simulink model "corr_mod_2_sim41_MI"  (R2021a)
settings: Solver=ode5  StartTime=0  StopTime=3  FixedStep=0.001  MaxStep=0.01  RelTol=1e-3  AbsTol=1e-3
values from neighbouring files (symbols this model uses):
  g = 9.81    [cipendco.m]
  l = 0.36    [cipendco.m]
  m = 0.23    [cipendco.m]
  M = 2.4    [cipendco.m]
settings Model: ExtModeTrigMode=oneshot  ExtModeArmWhenConnect=off  ExtModeAutoUpdateStatusClock=off  Creator=franckplestan  LastModifiedBy=Rodrigo
settings SolverCC: AutoScaleAbsTol=off  AlgebraicLoopSolver=TrustRegion
settings DataIOCC: SaveFormat=Array  SignalLoggingSaveFormat=ModelDataLogs  SaveOutput=off  ReturnWorkspaceOutputs=off
settings OptimizationCC: BooleanDataType=off  ExpressionDepthLimit=2147483647  InitFltsAndDblsToZero=on  LifeSpan=inf
settings DebuggingCC: SaveWithParameterizedLinksMsg=none  UnderspecifiedInitializationDetection=Classic  MergeDetectMultiDrivingBlocksExec=none  SignalResolutionControl=TryResolveAllWithWarning  MultiTaskDSMMsg=warning  MultiTaskCondExecSysMsg=none  FcnCallInpInsideContextMsg=warning  StateNameClashWarn=warning  SFUnexpectedBacktrackingDiag=warning  SFNoUnconditionalDefaultTransitionDiag=warning  SFExecutionAtInitializationDiag=none  SFMachineParentedDataDiag=warning  ArithmeticOperatorsInVariantConditions=warning
settings HardwareCC: ProdBitPerPointer=32  ProdBitPerSizeT=32  ProdBitPerPtrDiffT=32  ProdLargestAtomicFloat=None  ProdIntDivRoundTo=Undefined  ProdEndianess=Unspecified  ProdWordSize=32  ProdHWDeviceType=32-bit Generic  TargetUnknown=on
settings ModelReferenceCC: PropagateSignalLabelsOutOfModel=off
settings SFSimCC: SimUseLocalCustomCode=off  CustomCodeUndefinedFunction=UseInterfaceOnly
settings RTWCC: RTWUseLocalCustomCode=off
settings CodeAppCC: StateflowObjectComments=on
settings GRTTargetCC: TargetLangStandard=C89/C90 (ANSI)  ModelReferenceCompliant=off  ParMdlRefBuildCompliant=off  CompOptLevelCompliant=off  ConcurrentExecutionCompliant=off  CombineOutputUpdateFcns=off  MatFileLogging=off  MATLABClassNameForMDSCustomization=Simulink.SoftwareTarget.TargetSpecificTriggerConfigurationBase  GRTInterface=on
settings ConfigComp: CovMetricSettings=dw  CovSaveCumulativeToWorkspaceVar=on  CovSaveSingleToWorkspaceVar=on  CovExternalEMLEnable=off  CovSFcnEnable=off

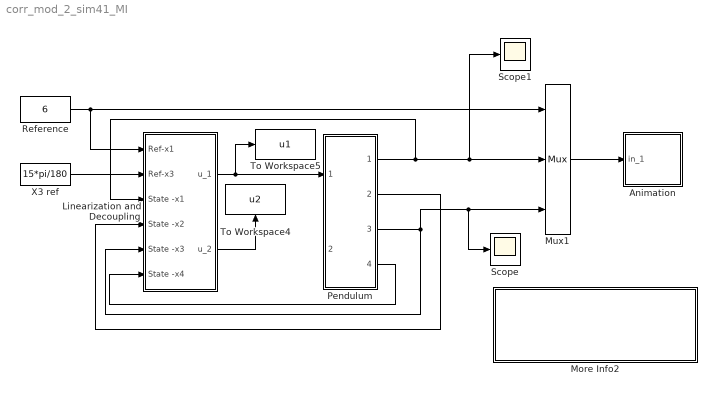
== system corr_mod_2_sim41_MI ==
  Animation : Subsystem  mask(Pendulum plot){RefBlock=Reference}
      mask prompts: RefBlock "DC reference signal block name:"
      mask help: Pendulum plot
      mask Help: Pendulum animation function using Handle graphics.
      mask Display: plot([-10 10],[0 0],[-2 -2 2 2],[0 1 1 0],[0 3],[1 5])
  Linearization and Decoupling : Subsystem
  More Info2 : Subsystem
      settings: OpenFcn=cipendco
      mask Display: disp('Init-File cipendco-doubleclick')
  Mux1 : Mux  Inputs=3
  Pendulum : Subsystem
  Reference : Constant  Value=6
  Scope : Scope
  Scope1 : Scope
  To Workspace4 : ToWorkspace  VariableName=u2  SampleTime=-1
  To Workspace5 : ToWorkspace  VariableName=u1  SampleTime=-1
  X3 ref : Constant  Value=15*pi/180
  wires:
  X3 ref/1 -> Linearization and Decoupling/2(Ref-x3)
  Pendulum/2(State-x2) -> Linearization and Decoupling/4(State -x2)
  Pendulum/4(State-x4) -> Linearization and Decoupling/6(State -x4)
  Linearization and Decoupling/2(u_2) -> To Workspace4/1
  Mux1/1 -> Animation/1(in_1)
  Pendulum/3(State-x3) -> Linearization and Decoupling/5(State -x3), Scope/1, Mux1/3
  Reference/1 -> Linearization and Decoupling/1(Ref-x1), Mux1/1
  Pendulum/1(State-x1) -> Linearization and Decoupling/3(State -x1), Scope1/1, Mux1/2
  Linearization and Decoupling/1(u_1) -> Pendulum/1(Input-u1), To Workspace5/1

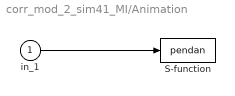
== system corr_mod_2_sim41_MI/Animation ==
  in_1 : Inport
  S-function : S-Function  FunctionName=pendan  Parameters=RefBlock  SFunctionDeploymentMode=off  EnableBusSupport=off
      settings: DeleteFcn=pendan([],[],[],'DeleteBlock');
  wires:
  in_1/1 -> S-function/1

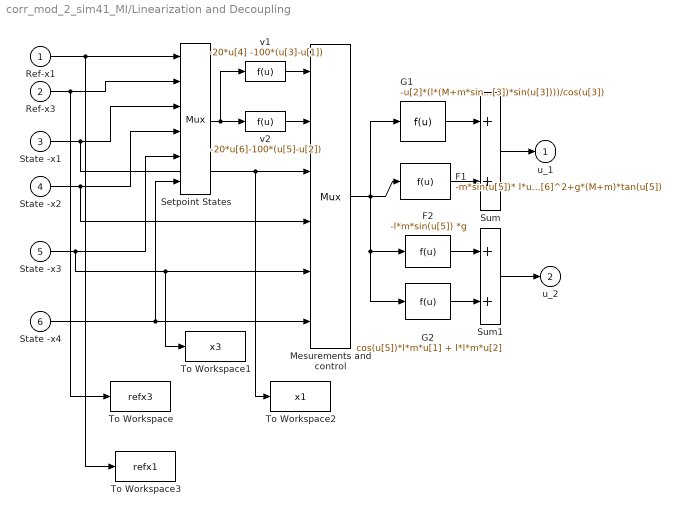
== system corr_mod_2_sim41_MI/Linearization and Decoupling ==
  Ref-x1 : Inport
  Ref-x3 : Inport  Port=2
  State -x1 : Inport  Port=3
  State -x2 : Inport  Port=4
  State -x3 : Inport  Port=5
  State -x4 : Inport  Port=6
  F1 : Fcn  Expr=-m*sin(u[5])* l*u[6]^2+g*(M+m)*tan(u[5])
  F2 : Fcn  Expr=-l*m*sin(u[5]) *g
  G1 : Fcn  Expr=-u[2]*(l*(M+m*sin(u[3])*sin(u[3])))/cos(u[3])
  G2 : Fcn  Expr=cos(u[5])*l*m*u[1] + l*l*m*u[2]
  Mesurements and control : Mux  Inputs=6
  Setpoint States : Mux  Inputs=6
  Sum : Sum  InputSameDT=on  SaturateOnIntegerOverflow=on  OutDataTypeStr=Inherit: Same as first input
  Sum1 : Sum  InputSameDT=on  SaturateOnIntegerOverflow=on  OutDataTypeStr=Inherit: Same as first input
  To Workspace : ToWorkspace  VariableName=refx3  SampleTime=-1
  To Workspace1 : ToWorkspace  VariableName=x3  SampleTime=-1
  To Workspace2 : ToWorkspace  VariableName=x1  SampleTime=-1
  To Workspace3 : ToWorkspace  VariableName=refx1  SampleTime=-1
  v1 : Fcn  Expr=-20*u[4] -100*(u[3]-u[1])
  v2 : Fcn  Expr=-20*u[6]-100*(u[5]-u[2])
  u_1 : Outport  VectorParamsAs1DForOutWhenUnconnected=off
  u_2 : Outport  Port=2  VectorParamsAs1DForOutWhenUnconnected=off
  wires:
  F1/1 -> Sum/2
  F2/1 -> Sum1/1
  G2/1 -> Sum1/2
  G1/1 -> Sum/1
  v1/1 -> Mesurements and control/1
  v2/1 -> Mesurements and control/2
  Mesurements and control/1 -> G1/1, F2/1, G2/1, F1/1
  Setpoint States/1 -> v1/1, v2/1
  State -x3/1 -> Setpoint States/5, Mesurements and control/5, To Workspace1/1
  State -x2/1 -> Setpoint States/4, Mesurements and control/4
  State -x1/1 -> Setpoint States/3, Mesurements and control/3, To Workspace2/1
  State -x4/1 -> Setpoint States/6, Mesurements and control/6
  Ref-x3/1 -> Setpoint States/2, To Workspace/1
  Ref-x1/1 -> Setpoint States/1, To Workspace3/1
  Sum/1 -> u_1/1
  Sum1/1 -> u_2/1

== system corr_mod_2_sim41_MI/More Info2 ==

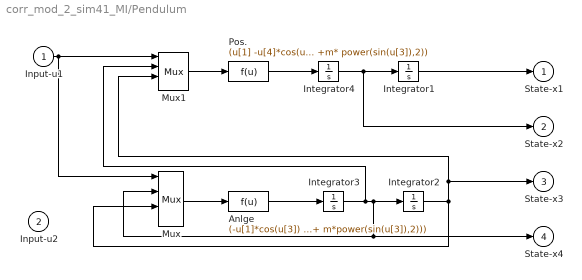
== system corr_mod_2_sim41_MI/Pendulum ==
  Input-u1 : Inport
  Input-u2 : Inport  Port=2
  Anlge : Fcn  Expr=(-u[1]*cos(u[3]) + u[4]*(M+m)/(m*l) + (M+m)*g*sin(u[3]) - m*l*power(u[2],2)*sin(u[3])*cos(u[3]))/(l*(M + m*power(sin(u[3]),2)))
  Integrator{1..4} (4 alike) : Integrator
  Mux : Mux
  Mux1 : Mux
  Pos. : Fcn  Expr=(u[1] -u[4]*cos(u[3])/l- m*g*sin(u[3])*cos(u[3]) + m*l*power(u[2],2)*sin(u[3]))/(M +m* power(sin(u[3]),2))
  State-x1 : Outport  VectorParamsAs1DForOutWhenUnconnected=off
  State-x2 : Outport  Port=2  VectorParamsAs1DForOutWhenUnconnected=off
  State-x3 : Outport  Port=3  VectorParamsAs1DForOutWhenUnconnected=off
  State-x4 : Outport  Port=4  VectorParamsAs1DForOutWhenUnconnected=off
  wires:
  Integrator2/1 -> Mux/3, Mux1/3, State-x3/1
  Input-u1/1 -> Mux1/1, Mux/1
  Integrator3/1 -> Integrator2/1, Mux/2, State-x4/1, Mux1/2
  Pos./1 -> Integrator4/1
  Mux1/1 -> Pos./1
  Mux/1 -> Anlge/1
  Anlge/1 -> Integrator3/1
  Integrator1/1 -> State-x1/1
  Integrator4/1 -> Integrator1/1, State-x2/1
